simulink model "original_decfir"  (R2012b)
settings: Solver=FixedStepDiscrete  SolverMode=SingleTasking  StartTime=0.0  StopTime=5000  FixedStep=1  RelTol=1e-3
libraries: xbsIndex_r4 x1499, xps_library x1, casper_library_misc x1
(part 1 of 15)
settings Model: Creator=paulp  LastModifiedBy=paulp
settings DataIOCC: LimitDataPoints=off
settings OptimizationCC: SimCompilerOptimization=On

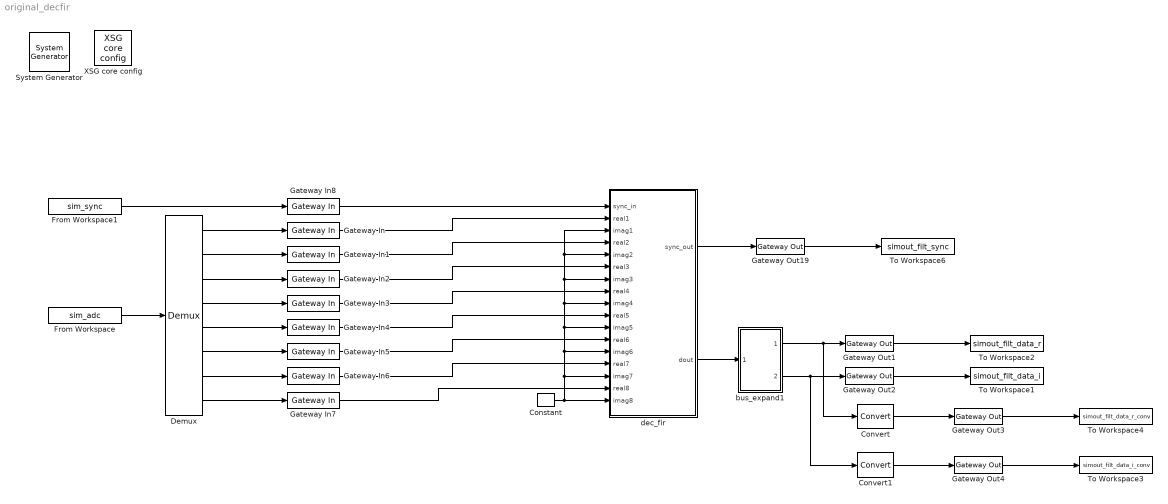
== system original_decfir ==
  " System Generator" : xbsIndex_r4/ System Generator  Tag=genX  xilinxfamily=virtex6  part=xc6vsx475t  speed=-1  package=ff1759  synthesis_tool=XST  clock_wrapper=Clock Enables  directory=./netlist  proj_type=Project Navigator  Synth_file=XST Defaults  Impl_file=ISE Defaults  testbench=off  simulink_period=1  sysclk_period=10  dcm_input_clock_period=10  incr_netlist=off  trim_vbits=Everywhere in SubSystem  dbl_ovrd=According to Block Masks  core_generation=According to Block Masks  run_coregen=off  deprecated_control=off  eval_field=0  block_type=sysgen
  Constant : xbsIndex_r4/Constant  const=0  gui_display_data_type=Fixed-point  arith_type=Signed (2's comp)  n_bits=10  bin_pt=9  preci_type=Single  exp_width=8  frac_width=24  explicit_period=on  period=1  equ=P=C  opselect=C  inp2=PCIN>>17  opr=+  inp1=P  carry=CIN  dbl_ovrd=off  block_type=constant
  Convert : xbsIndex_r4/Convert  gui_display_data_type=Fixed-point  arith_type="Signed  (2's comp)"  n_bits=10  bin_pt=9  float_type=Single  exp_bits=8  fraction_bits=24  quantization="Round  (unbiased: +/- Inf)"  overflow=Saturate  en=off  latency=0  dbl_ovrd=off  pipeline=off  block_type=convert
  Convert1 : xbsIndex_r4/Convert  gui_display_data_type=Fixed-point  arith_type="Signed  (2's comp)"  n_bits=10  bin_pt=9  float_type=Single  exp_bits=8  fraction_bits=24  quantization="Round  (unbiased: +/- Inf)"  overflow=Saturate  en=off  latency=0  dbl_ovrd=off  pipeline=off  block_type=convert
  Demux : Demux  Outputs=8
  From Workspace : FromWorkspace  VariableName=sim_adc  SampleTime=1  Interpolate=off  OutputAfterFinalValue=Setting to zero
  From Workspace1 : FromWorkspace  VariableName=sim_sync  SampleTime=1  Interpolate=off  OutputAfterFinalValue=Setting to zero
  Gateway In{,1..7} (8 alike) : xbsIndex_r4/Gateway In  gui_display_data_type=Fixed-point  arith_type="Signed  (2's comp)"  n_bits=10  bin_pt=9  preci_type=Single  exp_width=8  frac_width=24  quantization="Round  (unbiased: +/- Inf)"  overflow=Saturate  period=1  dbl_ovrd=off  timing_constraint=None  locs_specified=off  LOCs={}  UseAsADC=off  ADCChannel='1'  inherit_from_input=off  hdl_port=on  block_type=gatewayin
  Gateway In8 : xbsIndex_r4/Gateway In  gui_display_data_type=Boolean  arith_type=Boolean  n_bits=10  bin_pt=9  preci_type=Single  exp_width=8  frac_width=24  quantization="Round  (unbiased: +/- Inf)"  overflow=Saturate  period=1  dbl_ovrd=off  timing_constraint=None  locs_specified=off  LOCs={}  UseAsADC=off  ADCChannel='1'  inherit_from_input=off  hdl_port=on  block_type=gatewayin
  Gateway Out{1..4,19} (5 alike) : xbsIndex_r4/Gateway Out  inherit_from_input=off  hdl_port=off  timing_constraint=None  locs_specified=off  LOCs={}  UseAsDAC=off  DACChannel='1'  block_type=gatewayout
  To Workspace1 : ToWorkspace  VariableName=simout_filt_data_i  SampleTime=1  SaveFormat=Structure With Time
  To Workspace2 : ToWorkspace  VariableName=simout_filt_data_r  SampleTime=1  SaveFormat=Structure With Time
  To Workspace3 : ToWorkspace  VariableName=simout_filt_data_i_conv  SampleTime=1  SaveFormat=Structure With Time
  To Workspace4 : ToWorkspace  VariableName=simout_filt_data_r_conv  SampleTime=1  SaveFormat=Structure With Time
  To Workspace6 : ToWorkspace  VariableName=simout_filt_sync  SampleTime=1  SaveFormat=Structure With Time
  XSG core config : xps_library/XSG core config  Tag=xps:xsg  hw_sys=ROACH2:sx475t  clk_src=sys_clk  ROACH_clk_src=sys_clk  ROACH2_clk_src=sys_clk  MKDIG_clk_src=sys_clk  clk_rate=214  sample_period=1  synthesis_tool=XST
  bus_expand1 : Subsystem  AncestorBlock=casper_library_flow_control/bus_expand  mask(bus_expand){mode=divisions of equal size, outputNum=2, outputWidth=34, outputBinaryPt=24, outputArithmeticType=1, show_format=on, outputToWorkspace=off, variablePrefix=out, outputToModelAsWell=on}
      mask prompts: outputNum "Number of outputs:"; outputWidth "Output width:"; outputBinaryPt "Output binary point position:"; outputArithmeticType "Output arithmetic type (ufix=0, fix=1, bool=2):"; show_format "Print format string?"; outputToWorkspace "Output to workspace?"; variablePrefix "Variable name prefix:"; outputToModelAsWell "Output to model as well?"
      mask help:
      | Expands a 'bus' made using a bus_create or Xilinx
      | concat block.
      | The input will be divided into the specified number
      | of outputs with the specified arithmetic types.
      | Divisions are made from most significant bit.
      mask init:
      | bus_expand_init(gcb,...
      |     'mode', mode, ...
      |     'outputNum', outputNum, ...
      |     'outputWidth', outputWidth, ...
      |     'outputBinaryPt', outputBinaryPt, ...
      |     'outputArithmeticType', outputArithmeticType, ...
      |     'show_format', show_format, ...
      |     'outputToWorkspace', outputToWorkspace, ...
      |     'variablePrefix', variablePrefix, ...
      |     'outputToModelAsWell', outputToModelAsWell);
      settings: AttributesFormatString=2 outputs: f34.24,f34.24,
      mask TypeOptions mode: divisions of equal size | divisions of arbitrary size
      mask Callback mode: bus_expand_callback();
      mask Callback outputWidth: bus_expand_callback();
      mask Callback outputToWorkspace: bus_expand_callback();
  dec_fir : Subsystem  Tag=casper:dec_fir  AncestorBlock=casper_library_downconverter/dec_fir  mask(dec_fir){n_inputs=8, coeff=[0.000186138862561967	6.05689975479797e-05	8.98350104087398e-05	0.000110543122234595	0.000117904224321654	0.000108471378334606	8.09132221232553e-05	3.65582303050017e-05	-2.04120270065482e-05	-8.32013332028201e-05	-0.000143090017707379	-0.000190529266245985	-0.000216517472802937	-0.000214076824640890	-0.000179609377084864	-0.000113903548971865	-2.25891260939337e-05	8.40987722327739e-05	0.000192294648335760	0.000286154654418673	0.000350011326388348	0.000370758708830268	0.000340129079169465	0.000256501203398046	0.000125912076336999	-3.79699556913192e-05	-0.000215020597098951	-0.000380930590574616	-0.000510347724887166	-0.000580510267732332	-0.000574879092255934	-0.000486225854103541	-0.000318661611630257	-8.81975801603999e-05	0.000178391281207604	0.000446398633811858	0.000677461659587630	0.000834787008608676	0.000888649262107133	0.000821379908245343	0.000631067840528720	0.000333310900944456	-3.94154098318335e-05	-0.000440895364261436	-0.000816583986606924	-0.00111070634801855	-0.00127416276563883	-0.00127216409101298	-0.00109046866370132	-0.000739200022084217	-0.000253489505051640	0.000309415432622734	0.000876455210443800	0.00136785003024658	0.00170790291090728	0.00183610415695837	0.00171697165739811	0.00134711870763656	0.000758319656115441	1.58203380380529e-05	-0.000788238586137740	-0.00154572994613078	-0.00214656468763183	-0.00249408146197368	-0.00251972343912529	-0.00219486970517002	-0.00153793273500979	-0.000615363437934163	0.000464033612090709	0.00156117137403862	0.00252391176175991	0.00320741510313757	0.00349497892260422	0.00331647887793831	0.00266165338883929	0.00158599799575397	0.000207909436764838	-0.00130315557130700	-0.00274650585023830	-0.00391584232686132	-0.00462754200645335	-0.00474786541328700	-0.00421523988396043	-0.00305418148896349	-0.00137833093111497	0.000618598941726105	0.00268358902611891	0.00453478527075226	0.00589819831046895	0.00654606003089742	0.00633171920237173	0.00521606910972246	0.00328129539920438	0.000729148810282474	-0.00213716558118957	-0.00494625618186221	-0.00730362966306151	-0.00884344204529824	-0.00928051621840878	-0.00845573721601015	-0.00636831854562861	-0.00318968826340417	0.000744238830994179	0.00496307261864251	0.00891210060827213	0.0120177263229236	0.0137610719514846	0.0137511193525781	0.0117882493632991	0.00790963195912094	0.00240960151763348	-0.00416923242355217	-0.0110751157292765	-0.0174139397149507	-0.0222376853321542	-0.0246456483706254	-0.0238876286227442	-0.0194575143354574	-0.0111662667568517	0.000814814886236369	0.0159466703496291	0.0333532200898870	0.0518884159349622	0.0702336650993202	0.0870161869489056	0.100936348573347	0.110890810234390	0.116078553567419	0.116078553567419	0.110890810234390	0.100936348573347	0.0870161869489056	0.0702336650993202	0.0518884159349622	0.0333532200898870	0.0159466703496291	0.000814814886236369	-0.0111662667568517	-0.0194575143354574	-0.0238876286227442	-0.0246456483706254	-0.0222376853321542	-0.0174139397149507	-0.0110751157292765	-0.00416923242355217	0.00240960151763348	0.00790963195912094	0.0117882493632991	0.0137511193525781	0.0137610719514846	0.0120177263229236	0.00891210060827213	0.00496307261864251	0.000744238830994179	-0.00318968826340417	-0.00636831854562861	-0.00845573721601015	-0.00928051621840878	-0.00884344204529824	-0.00730362966306151	-0.00494625618186221	-0.00213716558118957	0.000729148810282474	0.00328129539920438	0.00521606910972246	0.00633171920237173	0.00654606003089742	0.00589819831046895	0.00453478527075226	0.00268358902611891	0.000618598941726105	-0.00137833093111497	-0.00305418148896349	-0.00421523988396043	-0.00474786541328700	-0.00462754200645335	-0.00391584232686132	-0.00274650585023830	-0.00130315557130700	0.000207909436764838	0.00158599799575397	0.00266165338883929	0.00331647887793831	0.00349497892260422	0.00320741510313757	0.00252391176175991	0.00156117137403862	0.000464033612090709	-0.000615363437934163	-0.00153793273500979	-0.00219486970517002	-0.00251972343912529	-0.00249408146197368	-0.00214656468763183	-0.00154572994613078	-0.000788238586137740	1.58203380380529e-05	0.000758319656115441	0.00134711870763656	0.00171697165739811	0.00183610415695837	0.00170790291090728	0.00136785003024658	0.000876455210443800	0.000309415432622734	-0.000253489505051640	-0.000739200022084217	-0.00109046866370132	-0.00127216409101298	-0.00127416276563883	-0.00111070634801855	-0.000816583986606924	-0.000440895364261436	-3.94154098318335e-05	0.000333310900944456	0.000631067840528720	0.000821379908245343	0.000888649262107133	0.000834787008608676	0.000677461659587630	0.000446398633811858	0.000178391281207604	-8.81975801603999e-05	-0.000318661611630257	-0.000486225854103541	-0.000574879092255934	-0.000580510267732332	-0.000510347724887166	-0.000380930590574616	-0.000215020597098951	-3.79699556913192e-05	0.000125912076336999	0.000256501203398046	0.000340129079169465	0.000370758708830268	0.000350011326388348	0.000286154654418673	0.000192294648335760	8.40987722327739e-05	-2.25891260939337e-05	-0.000113903548971865	-0.000179609377084864	-0.000214076824640890	-0.000216517472802937	-0.000190529266245985	-0.000143090017707379	-8.32013332028201e-05	-2.04120270065482e-05	3.65582303050017e-05	8.09132221232553e-05	0.000108471378334606	0.000117904224321654	0.000110543122234595	8.98350104087398e-05	6.05689975479797e-05	0.000186138862561967], n_bits=34, n_bits_bp=24, quantization=Round  (unbiased: +/- Inf), add_latency=1, mult_latency=2, conv_latency=2, coeff_bit_width=16, coeff_bin_pt=15, absorb_adders=off, adder_imp=Behavioral, lshift=0}
      mask prompts: n_inputs "Number of Parallel Streams"; coeff "Coefficients"; n_bits "Bit Width Out"; n_bits_bp "Bin Pt Out"; quantization "Quantization Behavior"; add_latency "Add Latency"; mult_latency "Mult Latency"; conv_latency "Convert latency"; coeff_bit_width "Coefficient bit width"; coeff_bin_pt "Coefficient binary point"; absorb_adders "Absorb adders into DSP slices"; adder_imp "Adder implementation"; lshift "Post adder-tree shift"
      mask help: FIR filter which can handle multiple time samples in parallel and decimates down to 1 time sample. If coefficients are symmetric, will automatically fold before multiplying.
      mask init:
      | dec_fir_init(gcb, ...
      |     'n_inputs', n_inputs, ...
      |     'coeff', coeff, ...
      |     'n_bits', n_bits, ...
      |     'n_bits_bp', n_bits_bp, ...
      |     'quantization', quantization, ...
      |     'add_latency', add_latency, ...
      |     'mult_latency', mult_latency, ...
      |     'conv_latency', conv_latency, ...
      |     'coeff_bit_width', coeff_bit_width, ...
      |     'coeff_bin_pt', coeff_bin_pt, ...
      |     'absorb_adders', absorb_adders, ...
      |     'adder_imp', adder_imp, ...
      |     'lshift', lshift);
      settings: AttributesFormatString=|
      | 256 taps
      | 34_24 r/i
      mask TypeOptions quantization: Truncate | Round  (unbiased: +/- Inf) | Round  (unbiased: Even Values)
      mask TypeOptions adder_imp: Behavioral | Fabric | DSP48
  wires:
  From Workspace/1 -> Demux/1
  From Workspace1/1 -> Gateway In8/1
  Demux/1 -> Gateway In/1
  Demux/2 -> Gateway In1/1
  Demux/3 -> Gateway In2/1
  Demux/4 -> Gateway In3/1
  Demux/5 -> Gateway In4/1
  Demux/6 -> Gateway In5/1
  Demux/7 -> Gateway In6/1
  Demux/8 -> Gateway In7/1
  Gateway In8/1 -> dec_fir/1(sync_in)
  Gateway In/1 -> dec_fir/2(real1)
  Gateway In1/1 -> dec_fir/4(real2)
  Gateway In2/1 -> dec_fir/6(real3)
  Gateway In3/1 -> dec_fir/8(real4)
  Gateway In4/1 -> dec_fir/10(real5)
  Gateway In5/1 -> dec_fir/12(real6)
  Gateway In6/1 -> dec_fir/14(real7)
  Gateway In7/1 -> dec_fir/16(real8)
  Constant/1 -> dec_fir/17(imag8), dec_fir/15(imag7), dec_fir/13(imag6), dec_fir/11(imag5), dec_fir/9(imag4), dec_fir/7(imag3), dec_fir/5(imag2), dec_fir/3(imag1)
  Gateway Out19/1 -> To Workspace6/1
  dec_fir/1(sync_out) -> Gateway Out19/1
  bus_expand1/1(msb_out2) -> Convert/1, Gateway Out1/1
  bus_expand1/2(lsb_out1) -> Convert1/1, Gateway Out2/1
  dec_fir/2(dout) -> bus_expand1/1(bus_in)
  Gateway Out1/1 -> To Workspace2/1
  Gateway Out2/1 -> To Workspace1/1
  Gateway Out3/1 -> To Workspace4/1
  Gateway Out4/1 -> To Workspace3/1
  Convert/1 -> Gateway Out3/1
  Convert1/1 -> Gateway Out4/1

== system original_decfir/bus_expand1 ==
  bus_in : Inport
  reinterpret1 : xbsIndex_r4/Reinterpret  force_arith_type=on  arith_type="Signed  (2's comp)"  force_bin_pt=on  bin_pt=24  block_type=reinterpret
  reinterpret2 : xbsIndex_r4/Reinterpret  force_arith_type=on  arith_type="Signed  (2's comp)"  force_bin_pt=on  bin_pt=24  block_type=reinterpret
  slice1 : xbsIndex_r4/Slice  nbits=34  boolean_output=off  mode=Upper Bit Location + Width  bit1=-34  base1=MSB of Input  bit0=0  base0=LSB of Input  dbl_ovrd=off  block_type=slice
  slice2 : xbsIndex_r4/Slice  nbits=34  boolean_output=off  mode=Upper Bit Location + Width  bit1=0  base1=MSB of Input  bit0=0  base0=LSB of Input  dbl_ovrd=off  block_type=slice
  msb_out2 : Outport
  lsb_out1 : Outport  Port=2
  wires:
  bus_in/1 -> slice2/1, slice1/1
  slice2/1 -> reinterpret2/1
  reinterpret2/1 -> msb_out2/1
  slice1/1 -> reinterpret1/1
  reinterpret1/1 -> lsb_out1/1
